simulink model "test_loopback_buf"  (Simulink 6.2)
settings: Solver=ode45  StartTime=0.0  StopTime=4000  RelTol=1e-3
undefined symbols (not defined in the file): Down, Up
libraries: xbsIndex_r3 x1383, xps_library x52, casper_library x37
(part 4 of 8)

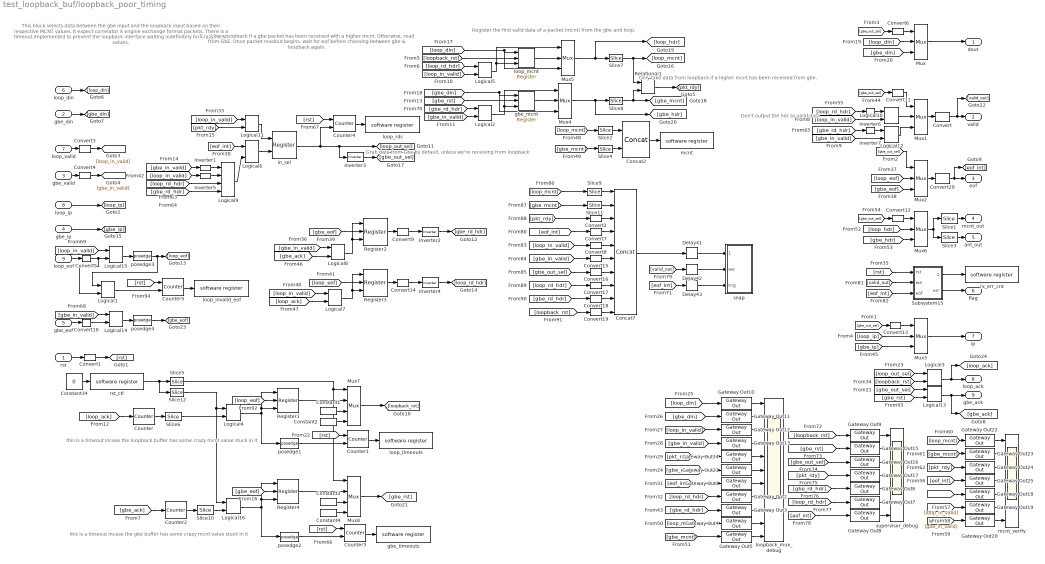
== system test_loopback_buf/loopback_poor_timing ==
  note: Read from loopback if a gbe packet
      | has been received with a higher mcnt.
      | Otherwise, read from GbE.
      | Once packet readout begins, wait for eof
      | before choosing between gbe & loopback again.
  note: Only take data from loopback
      | if a higher mcnt has been
      | received from gbe.
  note: This block selects data between the gbe input
      | and the loopback input based on their respective MCNT values.
      | It expect correlator X engine exchange format packets.
      |
      | There is a timeout implemented to prevent the loopback interface
      | waiting indefinitely for crazy MCNT values.
  note: Don't output the hdr
      | as valid data
  note: this is a timeout incase
      | the gbe buffer has
      | some crazy mcnt value stuck in it
  note: this is a timeout incase
      | the loopback buffer has
      | some crazy mcnt value stuck in it
  note: Grab data from
      | Gbe by default,
      | unless we're receiving
      | from loopback
  note: Register the first valid
      | data of a packet (mcnt)
      | from the gbe and loop.
  rst : Inport  Port=1  LatchInput=off
  gbe_din : Inport  Port=2  LatchInput=off
  gbe_valid : Inport  Port=3  LatchInput=off
  gbe_ip : Inport  Port=4  LatchInput=off
  gbe_eof : Inport  Port=5  LatchInput=off
  loop_din : Inport  Port=6  LatchInput=off
  loop_valid : Inport  Port=7  LatchInput=off
  loop_ip : Inport  Port=8  LatchInput=off
  loop_eof : Inport  Port=9  LatchInput=off
  Concat2 : xbsIndex_r3/Concat  num_inputs=2  explicit_period=off  period=1  dbl_ovrd=off
  Concat7 : xbsIndex_r3/Concat  num_inputs=10  explicit_period=off  period=1  dbl_ovrd=off
  Constant1 : xbsIndex_r3/Constant  const=0  equ=P=C  arith_type=Boolean  n_bits=1  bin_pt=0  opselect=C  inp2=PCIN>>17  opr=+  inp1=P  carry=CIN  iostate=0  explicit_period=on  period=1  dbl_ovrd=off
  Constant2 : xbsIndex_r3/Constant  const=1  equ=P=C  arith_type=Boolean  n_bits=1  bin_pt=0  opselect=C  inp2=PCIN>>17  opr=+  inp1=P  carry=CIN  iostate=0  explicit_period=on  period=1  dbl_ovrd=off
  Constant3 : xbsIndex_r3/Constant  const=0  equ=P=C  arith_type=Boolean  n_bits=1  bin_pt=0  opselect=C  inp2=PCIN>>17  opr=+  inp1=P  carry=CIN  iostate=0  explicit_period=on  period=1  dbl_ovrd=off
  Constant34 : Constant  Value=0
  Constant4 : xbsIndex_r3/Constant  const=1  equ=P=C  arith_type=Boolean  n_bits=1  bin_pt=0  opselect=C  inp2=PCIN>>17  opr=+  inp1=P  carry=CIN  iostate=0  explicit_period=on  period=1  dbl_ovrd=off
  Convert{,1,9,14,20} (5 alike) : xbsIndex_r3/Convert  arith_type=Boolean  n_bits=8  bin_pt=6  quantization=Truncate  overflow=Wrap  latency=0  explicit_period=off  period=1  dbl_ovrd=off  show_param=off  inserted_by_tool=off  pipeline=off
      settings: xl_area=[0, 0, 0, 0, 0, 0, 0]
  Convert{3..5,10} (4 alike) : xbsIndex_r3/Convert  arith_type=Boolean  n_bits=1  bin_pt=0  quantization=Truncate  overflow=Wrap  latency=0  explicit_period=on  period=1  dbl_ovrd=off  show_param=off  inserted_by_tool=off  pipeline=off
      settings: xl_area=[0, 0, 0, 0, 0, 0, 0]
  Convert{2,6..8,11..13,15..19} (12 alike) : xbsIndex_r3/Convert  arith_type=Unsigned  n_bits=1  bin_pt=0  quantization=Truncate  overflow=Wrap  latency=0  explicit_period=off  period=1  dbl_ovrd=off  show_param=off  inserted_by_tool=off  pipeline=off
      settings: xl_area=[0, 0, 0, 0, 0, 0, 0]
  Counter : xbsIndex_r3/Counter  cnt_type=Free Running  n_bits=timeout_bits+1  bin_pt=0  arith_type=Unsigned  start_count=0  cnt_to=Inf  cnt_by_val=1  operation=Up  explicit_period=off  period=1  load_pin=off  rst=on  en=off  dbl_ovrd=off  show_param=off  use_rpm=on  gen_core=off
      settings: xl_area=[0, 0, 0, 0, 0, 0, 0]
  Counter{1,3..5} (4 alike) : xbsIndex_r3/Counter  cnt_type=Free Running  n_bits=27  bin_pt=0  arith_type=Unsigned  start_count=0  cnt_to=Inf  cnt_by_val=1  operation=Up  explicit_period=off  period=1  load_pin=off  rst=on  en=on  dbl_ovrd=off  show_param=off  use_rpm=on  gen_core=off
      settings: xl_area=[0, 0, 0, 0, 0, 0, 0]
  Counter2 : xbsIndex_r3/Counter  cnt_type=Free Running  n_bits=timeout_bits+1  bin_pt=0  arith_type=Unsigned  start_count=0  cnt_to=Inf  cnt_by_val=1  operation=Up  explicit_period=off  period=1  load_pin=off  rst=on  en=off  dbl_ovrd=off  show_param=off  use_rpm=on  gen_core=off
      settings: xl_area=[0, 0, 0, 0, 0, 0, 0]
  Delay41 : xbsIndex_r3/Delay  latency=2  reg_retiming=on  explicit_period=on  period=1  en=off  accept_only_valid=off  init_zero=on  dbl_ovrd=off  show_param=off
      settings: xl_area=[0, 0, 0, 0, 0, 0, 0]
  Delay42 : xbsIndex_r3/Delay  latency=2  reg_retiming=on  explicit_period=on  period=1  en=off  accept_only_valid=off  init_zero=on  dbl_ovrd=off  show_param=off
      settings: xl_area=[0, 0, 0, 0, 0, 0, 0]
  Delay43 : xbsIndex_r3/Delay  latency=2  reg_retiming=on  explicit_period=on  period=1  en=off  accept_only_valid=off  init_zero=on  dbl_ovrd=off  show_param=off
      settings: xl_area=[0, 0, 0, 0, 0, 0, 0]
  Gateway Out{1..25} (25 alike) : xbsIndex_r3/Gateway Out  output_type=Double  nbits=8  bin_pt=6  arith_type=Boolean  quantization=Truncate  overflow=Wrap  hdl_port=on  timing_constraint=None  locs_specified=off  LOCs={}  needs_fixed_name=off  show_param=off
      settings: xl_area=[0, 0, 0, 0, 0, 0, 0]
  Inverter{1..7} (7 alike) : xbsIndex_r3/Inverter  latency=0  explicit_period=off  period=1  en=off  dbl_ovrd=off  show_param=off
      settings: xl_area=[0, 0, 0, 0, 0, 0, 0]
  Logical1 : xbsIndex_r3/Logical  logical_function=XOR  inputs=2  precision=Full  arith_type=Unsigned  n_bits=8  bin_pt=2  align_bp=on  latency=0  explicit_period=on  period=1  en=off  dbl_ovrd=off  show_param=off
      settings: xl_area=[0, 0, 0, 0, 0, 0, 0]
  Logical{7..8,10,14..15} (5 alike) : xbsIndex_r3/Logical  logical_function=AND  inputs=2  precision=Full  arith_type=Unsigned  n_bits=8  bin_pt=2  align_bp=on  latency=0  explicit_period=on  period=1  en=off  dbl_ovrd=off  show_param=off
      settings: xl_area=[0, 0, 0, 0, 0, 0, 0]
  Logical{2,5,11..12} (4 alike) : xbsIndex_r3/Logical  logical_function=AND  inputs=2  precision=Full  arith_type=Unsigned  n_bits=8  bin_pt=2  align_bp=on  latency=0  explicit_period=off  period=1  en=off  dbl_ovrd=off  show_param=off
      settings: xl_area=[0, 0, 0, 0, 0, 0, 0]
  Logical13 : xbsIndex_r3/Logical  logical_function=OR  inputs=2  precision=Full  arith_type=Unsigned  n_bits=8  bin_pt=2  align_bp=on  latency=0  explicit_period=off  period=1  en=off  dbl_ovrd=off  show_param=off
      settings: xl_area=[0, 0, 0, 0, 0, 0, 0]
  Logical16 : xbsIndex_r3/Logical  logical_function=OR  inputs=2  precision=Full  arith_type=Unsigned  n_bits=8  bin_pt=2  align_bp=on  latency=0  explicit_period=on  period=1  en=off  dbl_ovrd=off  show_param=off
      settings: xl_area=[0, 0, 0, 0, 0, 0, 0]
  Logical3 : xbsIndex_r3/Logical  logical_function=OR  inputs=2  precision=Full  arith_type=Unsigned  n_bits=8  bin_pt=2  align_bp=on  latency=0  explicit_period=off  period=1  en=off  dbl_ovrd=off  show_param=off
      settings: xl_area=[0, 0, 0, 0, 0, 0, 0]
  Logical4 : xbsIndex_r3/Logical  logical_function=OR  inputs=2  precision=Full  arith_type=Unsigned  n_bits=8  bin_pt=2  align_bp=on  latency=0  explicit_period=on  period=1  en=off  dbl_ovrd=off  show_param=off
      settings: xl_area=[0, 0, 0, 0, 0, 0, 0]
  Logical6 : xbsIndex_r3/Logical  logical_function=OR  inputs=2  precision=Full  arith_type=Unsigned  n_bits=8  bin_pt=2  align_bp=on  latency=0  explicit_period=off  period=1  en=off  dbl_ovrd=off  show_param=off
      settings: xl_area=[0, 0, 0, 0, 0, 0, 0]
  Logical9 : xbsIndex_r3/Logical  logical_function=AND  inputs=4  precision=Full  arith_type=Unsigned  n_bits=8  bin_pt=2  align_bp=on  latency=0  explicit_period=on  period=1  en=off  dbl_ovrd=off  show_param=off
      settings: xl_area=[0, 0, 0, 0, 0, 0, 0]
  Mux{,1,3..6} (6 alike) : xbsIndex_r3/Mux  inputs=2  precision=Full  arith_type="Signed  (2's comp)"  n_bits=8  bin_pt=2  quantization=Truncate  overflow=Wrap  latency=0  explicit_period=off  period=1  en=off  dbl_ovrd=off  show_param=off  mux_type=off  use_rpm=off  gen_core=off
      settings: xl_area=[0, 0, 0, 0, 0, 0, 0]
  Mux2 : xbsIndex_r3/Mux  inputs=2  precision=Full  arith_type="Signed  (2's comp)"  n_bits=8  bin_pt=2  quantization=Truncate  overflow=Wrap  latency=0  explicit_period=on  period=1  en=off  dbl_ovrd=off  show_param=off  mux_type=off  use_rpm=off  gen_core=off
      settings: xl_area=[0, 0, 0, 0, 0, 0, 0]
  Mux7 : xbsIndex_r3/Mux  inputs=3  precision=Full  arith_type="Signed  (2's comp)"  n_bits=8  bin_pt=2  quantization=Truncate  overflow=Wrap  latency=0  explicit_period=off  period=1  en=off  dbl_ovrd=off  show_param=off  mux_type=off  use_rpm=off  gen_core=off
      settings: xl_area=[0, 0, 0, 0, 0, 0, 0]
  Mux8 : xbsIndex_r3/Mux  inputs=3  precision=Full  arith_type="Signed  (2's comp)"  n_bits=8  bin_pt=2  quantization=Truncate  overflow=Wrap  latency=0  explicit_period=off  period=1  en=off  dbl_ovrd=off  show_param=off  mux_type=off  use_rpm=off  gen_core=off
      settings: xl_area=[0, 0, 0, 0, 0, 0, 0]
  Register{1..4} (4 alike) : xbsIndex_r3/Register  init=0  reg_only_valid=off  explicit_period=on  period=1  rst=on  en=on  out_en=off  dbl_ovrd=off  show_param=off
      settings: xl_area=[0, 0, 0, 0, 0, 0, 0]
  Relational1 : xbsIndex_r3/Relational  mode=a<b  latency=0  explicit_period=off  period=1  en=off  dbl_ovrd=off  show_param=off
      settings: xl_area=[0, 0, 0, 0, 0, 0, 0]
  Slice1 : xbsIndex_r3/Slice  mode=Lower Bit Location + Width  nbits=48  bit1=0  base1=MSB of Input  bit0=16  base0=LSB of Input  boolean_output=off  explicit_period=off  period=1  dbl_ovrd=off
  Slice10 : xbsIndex_r3/Slice  mode=Upper Bit Location + Width  nbits=1  bit1=0  base1=MSB of Input  bit0=1  base0=LSB of Input  boolean_output=on  explicit_period=off  period=1  dbl_ovrd=off
  Slice11 : xbsIndex_r3/Slice  mode=Lower Bit Location + Width  nbits=12  bit1=0  base1=MSB of Input  bit0=0  base0=LSB of Input  boolean_output=off  explicit_period=off  period=1  dbl_ovrd=off
  Slice12 : xbsIndex_r3/Slice  mode=Lower Bit Location + Width  nbits=1  bit1=0  base1=MSB of Input  bit0=0  base0=LSB of Input  boolean_output=on  explicit_period=off  period=1  dbl_ovrd=off
  Slice2 : xbsIndex_r3/Slice  mode=Lower Bit Location + Width  nbits=16  bit1=0  base1=MSB of Input  bit0=0  base0=LSB of Input  boolean_output=off  explicit_period=off  period=1  dbl_ovrd=off
  Slice3 : xbsIndex_r3/Slice  mode=Lower Bit Location + Width  nbits=16  bit1=0  base1=MSB of Input  bit0=0  base0=LSB of Input  boolean_output=off  explicit_period=off  period=1  dbl_ovrd=off
  Slice4 : xbsIndex_r3/Slice  mode=Lower Bit Location + Width  nbits=16  bit1=0  base1=MSB of Input  bit0=0  base0=LSB of Input  boolean_output=off  explicit_period=off  period=1  dbl_ovrd=off
  Slice5 : xbsIndex_r3/Slice  mode=Lower Bit Location + Width  nbits=2  bit1=0  base1=MSB of Input  bit0=1  base0=LSB of Input  boolean_output=off  explicit_period=off  period=1  dbl_ovrd=off
  Slice6 : xbsIndex_r3/Slice  mode=Upper Bit Location + Width  nbits=1  bit1=0  base1=MSB of Input  bit0=1  base0=LSB of Input  boolean_output=on  explicit_period=off  period=1  dbl_ovrd=off
  Slice7 : xbsIndex_r3/Slice  mode=Upper Bit Location + Width  nbits=48  bit1=0  base1=MSB of Input  bit0=0  base0=LSB of Input  boolean_output=off  explicit_period=off  period=1  dbl_ovrd=off
  Slice8 : xbsIndex_r3/Slice  mode=Upper Bit Location + Width  nbits=48  bit1=0  base1=MSB of Input  bit0=0  base0=LSB of Input  boolean_output=off  explicit_period=off  period=1  dbl_ovrd=off
  Slice9 : xbsIndex_r3/Slice  mode=Lower Bit Location + Width  nbits=12  bit1=0  base1=MSB of Input  bit0=0  base0=LSB of Input  boolean_output=off  explicit_period=off  period=1  dbl_ovrd=off
  Subsystem15 : Subsystem  mask{payload_len=payload_len}
      mask init:
      | fmtstr = sprintf('Payload Length: %d', payload_len);
      | set_param(gcb, 'AttributesFormatString', fmtstr);
      settings: AttributesFormatString=Payload Length: 50
  gbe_mcnt : xbsIndex_r3/Register  init=0  reg_only_valid=off  explicit_period=on  period=1  rst=on  en=on  out_en=off  dbl_ovrd=off  show_param=off
      settings: xl_area=[0, 0, 0, 0, 0, 0, 0]
  gbe_timeouts : xps_library/software register  Tag=xps:sw_reg  io_dir=To Processor  arith_type=Unsigned  bitwidth=32  bin_pt=0  sample_period=1  gw_name=test_loopback_buf_loopback_poor_timing_gbe_timeouts_user_data_in
  in_sel : xbsIndex_r3/Register  init=0  reg_only_valid=off  explicit_period=on  period=1  rst=off  en=on  out_en=off  dbl_ovrd=off  show_param=off
      settings: xl_area=[0, 0, 0, 0, 0, 0, 0]
  loop_invalid_eof : xps_library/software register  Tag=xps:sw_reg  io_dir=To Processor  arith_type=Unsigned  bitwidth=32  bin_pt=0  sample_period=1  gw_name=test_loopback_buf_loopback_poor_timing_loop_invalid_eof_user_data_in
  loop_mcnt : xbsIndex_r3/Register  init=0  reg_only_valid=off  explicit_period=on  period=1  rst=on  en=on  out_en=off  dbl_ovrd=off  show_param=off
      settings: xl_area=[0, 0, 0, 0, 0, 0, 0]
  loop_rds : xps_library/software register  Tag=xps:sw_reg  io_dir=To Processor  arith_type=Unsigned  bitwidth=32  bin_pt=0  sample_period=1  gw_name=test_loopback_buf_loopback_poor_timing_loop_rds_user_data_in
  loop_timeouts : xps_library/software register  Tag=xps:sw_reg  io_dir=To Processor  arith_type=Unsigned  bitwidth=32  bin_pt=0  sample_period=1  gw_name=test_loopback_buf_loopback_poor_timing_loop_timeouts_user_data_in
  loopback_mux_debug : Scope  NumInputPorts=11
      settings: YMin=300~190.95~0~0.95~0.95~-1~-1~-1~-5~-5~-5  YMax=525~211.05~1~1.05~1.05~1~1~1~5~5~5  SaveName=ScopeData7
  mcnt : xps_library/software register  Tag=xps:sw_reg  io_dir=To Processor  arith_type=Unsigned  bitwidth=32  bin_pt=0  sample_period=1  gw_name=test_loopback_buf_loopback_poor_timing_mcnt_user_data_in
  mcnt_verify : Scope  NumInputPorts=7
      settings: YMin=300~190.95~0~-5~-5~-5~-5  YMax=525~211.05~1~5~5~5~5  SaveName=ScopeData2
  posedge{1..4} (4 alike) : casper_library/Misc/posedge  Tag=Rising Edge Detector
  rst_ctl : xps_library/software register  Tag=xps:sw_reg  io_dir=From Processor  arith_type=Unsigned  bitwidth=32  bin_pt=0  sample_period=1  gw_name=test_loopback_buf_loopback_poor_timing_rst_ctl_user_data_out
  rx_err_cnt : xps_library/software register  Tag=xps:sw_reg  io_dir=To Processor  arith_type=Unsigned  bitwidth=32  bin_pt=0  sample_period=1  gw_name=test_loopback_buf_loopback_poor_timing_rx_err_cnt_user_data_in
  snap : Subsystem  mask{nsamples=12}
      mask prompts: nsamples "Number of Samples (2^?)"
  supervisor_debug : Scope  NumInputPorts=7
      settings: YMin=300~190.95~0~-5~-5~-5~-5  YMax=525~211.05~1~5~5~5~5  SaveName=ScopeData18
  dout : Outport
  valid : Outport  Port=2
  eof : Outport  Port=3
  mcnt_out : Outport  Port=4
  ant_out : Outport  Port=5
  flag : Outport  Port=6
  ip : Outport  Port=7
  loop_ack : Outport  Port=8
  gbe_ack : Outport  Port=9
  wires:
  Mux/1 -> dout/1
  Mux1/1 -> Convert/1
  Mux2/1 -> Convert20/1
  gbe_valid/1 -> Convert4/1
  loop_valid/1 -> Convert3/1
  Convert/1 -> valid/1, [valid_out]
  Slice2/1 -> Concat2/1
  Slice4/1 -> Concat2/2
  Concat2/1 -> mcnt/1
  Convert6/1 -> Mux/1
  [gbe_out_sel] -> Convert6/1
  [gbe_out_sel] -> Mux2/1
  Gateway Out12/1 -> loopback_mux_debug/3
  Gateway Out13/1 -> loopback_mux_debug/4
  Gateway Out14/1 -> loopback_mux_debug/5
  Gateway Out21/1 -> loopback_mux_debug/6
  Convert3/1 -> [loop_in_valid]
  Convert4/1 -> [gbe_in_valid]
  Relational1/1 -> [pkt_rdy]
  loop_din/1 -> [loop_din]
  gbe_din/1 -> [gbe_din]
  [loop_din] -> Mux/2
  [gbe_din] -> Mux/3
  [gbe_din] -> Gateway Out11/1
  [loop_din] -> Gateway Out10/1
  [loop_in_valid] -> Gateway Out12/1
  [gbe_in_valid] -> Gateway Out13/1
  [gbe_out_sel] -> Gateway Out21/1
  [pkt_rdy] -> Gateway Out14/1
  Gateway Out1/1 -> loopback_mux_debug/7
  [eof_int] -> Gateway Out1/1
  [loop_rd_hdr] -> Gateway Out2/1
  Gateway Out2/1 -> loopback_mux_debug/8
  [loop_eof] -> Mux2/2
  loop_eof/1 -> Convert5/1
  gbe_eof/1 -> Convert10/1
  [gbe_eof] -> Mux2/3
  Gateway Out3/1 -> loopback_mux_debug/9
  [gbe_rd_hdr] -> Gateway Out3/1
  [gbe_out_sel] -> Convert11/1
  Convert11/1 -> Mux1/1
  loop_ip/1 -> [loop_ip]
  gbe_ip/1 -> [gbe_ip]
  Mux3/1 -> ip/1
  [loop_ip] -> Mux3/2
  [gbe_ip] -> Mux3/3
  [gbe_out_sel] -> Convert13/1
  Convert13/1 -> Mux3/1
  [loop_mcnt] -> Slice2/1
  [gbe_mcnt] -> Slice4/1
  Gateway Out10/1 -> loopback_mux_debug/1
  Gateway Out11/1 -> loopback_mux_debug/2
  Gateway Out4/1 -> loopback_mux_debug/10
  Gateway Out5/1 -> loopback_mux_debug/11
  [loop_mcnt] -> Gateway Out4/1
  [gbe_mcnt] -> Gateway Out5/1
  Gateway Out24/1 -> mcnt_verify/3
  Gateway Out22/1 -> mcnt_verify/1
  Gateway Out23/1 -> mcnt_verify/2
  Gateway Out25/1 -> mcnt_verify/4
  Gateway Out18/1 -> mcnt_verify/5
  Gateway Out19/1 -> mcnt_verify/6
  Gateway Out20/1 -> mcnt_verify/7
  [gbe_out_sel] -> Gateway Out20/1
  [gbe_in_valid] -> Gateway Out19/1
  [loop_in_valid] -> Gateway Out18/1
  [eof_int] -> Gateway Out25/1
  [loop_mcnt] -> Gateway Out22/1
  [gbe_mcnt] -> Gateway Out23/1
  [pkt_rdy] -> Gateway Out24/1
  Mux4/1 -> Slice8/1, [gbe_hdr]
  Mux5/1 -> Slice7/1, [loop_hdr]
  Slice7/1 -> Relational1/1, [loop_mcnt]
  Slice8/1 -> Relational1/2, [gbe_mcnt]
  Slice1/1 -> mcnt_out/1
  Slice3/1 -> ant_out/1
  Convert12/1 -> Mux6/1
  [gbe_out_sel] -> Convert12/1
  [loop_hdr] -> Mux6/2
  [gbe_hdr] -> Mux6/3
  Mux6/1 -> Slice1/1, Slice3/1
  Inverter6/1 -> Logical10/1
  Logical10/1 -> Mux1/2
  [loop_in_valid] -> Logical10/2
  [loop_rd_hdr] -> Inverter6/1
  [gbe_rd_hdr] -> Inverter7/1
  [gbe_in_valid] -> Logical12/2
  Logical12/1 -> Mux1/3
  Inverter7/1 -> Logical12/1
  Counter2/1 -> Slice10/1
  [gbe_ack] -> Counter2/1
  [rst] -> Counter3/1
  Counter3/1 -> gbe_timeouts/1
  Logical16/1 -> Register4/1, Register4/3, posedge2/1
  Logical14/1 -> posedge4/1
  Logical15/1 -> posedge3/1
  Convert5/1 -> Logical15/2, Logical1/2
  Convert10/1 -> Logical14/2
  [gbe_in_valid] -> Logical14/1
  [loop_in_valid] -> Logical15/1
  Slice10/1 -> Logical16/2
  Gateway Out16/1 -> supervisor_debug/3
  Gateway Out9/1 -> supervisor_debug/1
  Gateway Out15/1 -> supervisor_debug/2
  Gateway Out17/1 -> supervisor_debug/4
  Gateway Out6/1 -> supervisor_debug/5
  Gateway Out7/1 -> supervisor_debug/6
  Gateway Out8/1 -> supervisor_debug/7
  [loopback_rst] -> Gateway Out9/1
  [gbe_rst] -> Gateway Out15/1
  [gbe_out_sel] -> Gateway Out16/1
  [pkt_rdy] -> Gateway Out17/1
  [gbe_rd_hdr] -> Gateway Out6/1
  [loop_rd_hdr] -> Gateway Out7/1
  [eof_int] -> Gateway Out8/1
  Logical3/1 -> loop_ack/1, [loop_ack]
  Logical13/1 -> gbe_ack/1, [gbe_ack]
  rst/1 -> Convert1/1
  Subsystem15/1(err_cnt) -> rx_err_cnt/1
  Subsystem15/2(err) -> flag/1
  [rst] -> Subsystem15/1(rst)
  [valid_out] -> Subsystem15/2(we)
  [eof_int] -> Subsystem15/3(eof)
  Counter/1 -> Slice6/1
  Slice6/1 -> Logical4/2
  [loop_ack] -> Counter/1
  [rst] -> Counter1/1
  Counter1/1 -> loop_timeouts/1
  Logical4/1 -> Register1/1, Register1/3, posedge1/1
  [pkt_rdy] -> Logical11/2
  [eof_int] -> Logical6/1
  Inverter3/1 -> [gbe_out_sel]
  in_sel/1 -> Inverter3/1, [loop_out_sel], Counter4/2
  Logical6/1 -> in_sel/2
  [loop_in_valid] -> Logical11/1
  Register2/1 -> Convert9/1
  Convert9/1 -> Inverter2/1
  Inverter2/1 -> [gbe_rd_hdr]
  [gbe_eof] -> Register2/2
  Register3/1 -> Convert14/1
  Convert14/1 -> Inverter4/1
  Inverter4/1 -> [loop_rd_hdr]
  [loop_eof] -> Register3/2
  Logical11/1 -> in_sel/1
  Logical8/1 -> Register2/1, Register2/3
  [gbe_in_valid] -> Logical8/1
  [gbe_ack] -> Logical8/2
  Logical7/1 -> Register3/1, Register3/3
  [loop_in_valid] -> Logical7/1
  [loop_ack] -> Logical7/2
  [gbe_in_valid] -> Inverter1/1
  [loop_in_valid] -> Inverter5/1
  Logical9/1 -> Logical6/2
  Inverter1/1 -> Logical9/1
  Inverter5/1 -> Logical9/2
  [loop_rd_hdr] -> Logical9/3
  [gbe_rd_hdr] -> Logical9/4
  gbe_mcnt/1 -> Mux4/2
  loop_mcnt/1 -> Mux5/2
  Logical2/1 -> gbe_mcnt/3, Mux4/1
  Logical5/1 -> Mux5/1, loop_mcnt/3
  [loop_rd_hdr] -> Logical5/1
  [gbe_rd_hdr] -> Logical2/1
  [loop_in_valid] -> Logical5/2
  [gbe_in_valid] -> Logical2/2
  [loop_din] -> loop_mcnt/1, Mux5/3
  [gbe_din] -> gbe_mcnt/1, Mux4/3
  Concat7/1 -> Delay41/1
  Delay42/1 -> snap/2(we)
  Delay43/1 -> snap/3(trig)
  Delay41/1 -> snap/1(data_in)
  [valid_out] -> Delay42/1
  [eof_int] -> Delay43/1
  [loop_mcnt] -> Slice9/1
  [gbe_mcnt] -> Slice11/1
  Slice9/1 -> Concat7/1
  Slice11/1 -> Concat7/2
  [pkt_rdy] -> Convert2/1
  [eof_int] -> Convert7/1
  [loop_in_valid] -> Convert8/1
  [gbe_in_valid] -> Convert15/1
  [gbe_out_sel] -> Convert16/1
  [loop_rd_hdr] -> Convert17/1
  [gbe_rd_hdr] -> Convert18/1
  [loopback_rst] -> Convert19/1
  [loop_eof] -> Register1/2
  [gbe_eof] -> Register4/2
  [loop_out_sel] -> Logical3/1
  [gbe_out_sel] -> Logical13/1
  [loopback_rst] -> Logical3/2
  [gbe_rst] -> Logical13/2
  Mux7/1 -> [loopback_rst]
  Register1/1 -> Mux7/2
  Mux8/1 -> [gbe_rst]
  Register4/1 -> Mux8/2
  Constant1/1 -> Mux7/3
  Constant34/1 -> rst_ctl/1
  rst_ctl/1 -> Slice5/1, Slice12/1
  Slice5/1 -> Mux7/1, Mux8/1
  Convert1/1 -> [rst]
  Slice12/1 -> Logical4/1, Logical16/1
  [loopback_rst] -> loop_mcnt/2
  [gbe_rst] -> gbe_mcnt/2
  Convert2/1 -> Concat7/3
  Convert7/1 -> Concat7/4
  Convert8/1 -> Concat7/5
  Convert15/1 -> Concat7/6
  Convert16/1 -> Concat7/7
  Convert17/1 -> Concat7/8
  Convert18/1 -> Concat7/9
  Convert19/1 -> Concat7/10
  Counter4/1 -> loop_rds/1
  [rst] -> Counter4/1
  Convert20/1 -> [eof_int], eof/1
  posedge1/1 -> Counter1/2
  posedge2/1 -> Counter3/2
  posedge3/1 -> [loop_eof], Logical1/1
  posedge4/1 -> [gbe_eof]
  [rst] -> Counter5/1
  Counter5/1 -> loop_invalid_eof/1
  Logical1/1 -> Counter5/2
  Constant2/1 -> Mux7/4
  Constant3/1 -> Mux8/3
  Constant4/1 -> Mux8/4

== system test_loopback_buf/mux_pkts_orig ==
  note: Read from loopback if a gbe packet
      | has been received with a higher mcnt.
      | Otherwise, wait until gbe has one ready.
      | Once packet readout begins, wait for eof
      | before choosing between gbe & loopback again.
  note: Register the first valid
      | data of a packet (mcnt)
      | from the gbe.
  note: Only take data from loopback
      | if a higher mcnt has been
      | received from gbe.
  gbe_din : Inport  Port=1  LatchInput=off
  gbe_valid : Inport  Port=2  LatchInput=off
  gbe_eof : Inport  Port=3  LatchInput=off
  loop_din : Inport  Port=4  LatchInput=off
  loop_valid : Inport  Port=5  LatchInput=off
  loop_eof : Inport  Port=6  LatchInput=off
  Concat2 : xbsIndex_r3/Concat  num_inputs=2  explicit_period=off  period=1  dbl_ovrd=off
  Constant1 : Constant  Value=0
  Convert : xbsIndex_r3/Convert  arith_type=Boolean  n_bits=8  bin_pt=6  quantization=Truncate  overflow=Wrap  latency=0  explicit_period=off  period=1  dbl_ovrd=off  show_param=off  inserted_by_tool=off  pipeline=off
      settings: xl_area=[0, 0, 0, 0, 0, 0, 0]
  Convert1 : xbsIndex_r3/Convert  arith_type=Boolean  n_bits=8  bin_pt=6  quantization=Truncate  overflow=Wrap  latency=0  explicit_period=off  period=1  dbl_ovrd=off  show_param=off  inserted_by_tool=off  pipeline=off
      settings: xl_area=[0, 0, 0, 0, 0, 0, 0]
  Convert2 : xbsIndex_r3/Convert  arith_type=Boolean  n_bits=8  bin_pt=6  quantization=Truncate  overflow=Wrap  latency=0  explicit_period=off  period=1  dbl_ovrd=off  show_param=off  inserted_by_tool=off  pipeline=off
      settings: xl_area=[0, 0, 0, 0, 0, 0, 0]
  Convert{4..5,7..8} (4 alike) : xbsIndex_r3/Convert  arith_type=Boolean  n_bits=1  bin_pt=0  quantization=Truncate  overflow=Wrap  latency=0  explicit_period=on  period=1  dbl_ovrd=off  show_param=off  inserted_by_tool=off  pipeline=off
      settings: xl_area=[0, 0, 0, 0, 0, 0, 0]
  Convert6 : xbsIndex_r3/Convert  arith_type=Unsigned  n_bits=1  bin_pt=0  quantization=Truncate  overflow=Wrap  latency=0  explicit_period=off  period=1  dbl_ovrd=off  show_param=off  inserted_by_tool=off  pipeline=off
      settings: xl_area=[0, 0, 0, 0, 0, 0, 0]
  Delay1 : xbsIndex_r3/Delay  latency=1  reg_retiming=off  explicit_period=off  period=1  en=off  accept_only_valid=off  init_zero=on  dbl_ovrd=off  show_param=off
      settings: xl_area=[0, 0, 0, 0, 0, 0, 0]
  Inverter2 : xbsIndex_r3/Inverter  Orientation=left  latency=0  explicit_period=off  period=1  en=off  dbl_ovrd=off  show_param=off
      settings: xl_area=[0, 0, 0, 0, 0, 0, 0]
  Logical : xbsIndex_r3/Logical  logical_function=OR  inputs=2  precision=Full  arith_type=Unsigned  n_bits=8  bin_pt=2  align_bp=on  latency=0  explicit_period=off  period=1  en=off  dbl_ovrd=off  show_param=off
      settings: xl_area=[0, 0, 0, 0, 0, 0, 0]
  Logical{1..5,7..8} (7 alike) : xbsIndex_r3/Logical  logical_function=AND  inputs=2  precision=Full  arith_type=Unsigned  n_bits=8  bin_pt=2  align_bp=on  latency=0  explicit_period=off  period=1  en=off  dbl_ovrd=off  show_param=off
      settings: xl_area=[0, 0, 0, 0, 0, 0, 0]
  Logical9 : xbsIndex_r3/Logical  logical_function=OR  inputs=2  precision=Full  arith_type=Unsigned  n_bits=8  bin_pt=2  align_bp=on  latency=1  explicit_period=off  period=1  en=off  dbl_ovrd=off  show_param=off
      settings: xl_area=[0, 0, 0, 0, 0, 0, 0]
  Mux : xbsIndex_r3/Mux  inputs=2  precision=Full  arith_type="Signed  (2's comp)"  n_bits=8  bin_pt=2  quantization=Truncate  overflow=Wrap  latency=1  explicit_period=off  period=1  en=off  dbl_ovrd=off  show_param=off  mux_type=off  use_rpm=off  gen_core=off
      settings: xl_area=[0, 0, 0, 0, 0, 0, 0]
  Mux2 : xbsIndex_r3/Mux  inputs=2  precision=Full  arith_type="Signed  (2's comp)"  n_bits=8  bin_pt=2  quantization=Truncate  overflow=Wrap  latency=0  explicit_period=off  period=1  en=off  dbl_ovrd=off  show_param=off  mux_type=off  use_rpm=off  gen_core=off
      settings: xl_area=[0, 0, 0, 0, 0, 0, 0]
  Relational1 : xbsIndex_r3/Relational  mode=a<=b  latency=1  explicit_period=off  period=1  en=off  dbl_ovrd=off  show_param=off
      settings: xl_area=[0, 0, 0, 0, 0, 0, 0]
  Slice : xbsIndex_r3/Slice  mode=Lower Bit Location + Width  nbits=1  bit1=0  base1=MSB of Input  bit0=1  base0=LSB of Input  boolean_output=off  explicit_period=off  period=1  dbl_ovrd=off
  Slice1 : xbsIndex_r3/Slice  mode=Upper Bit Location + Width  nbits=48  bit1=0  base1=MSB of Input  bit0=0  base0=LSB of Input  boolean_output=off  explicit_period=off  period=1  dbl_ovrd=off
  Slice2 : xbsIndex_r3/Slice  mode=Lower Bit Location + Width  nbits=16  bit1=0  base1=MSB of Input  bit0=0  base0=LSB of Input  boolean_output=off  explicit_period=off  period=1  dbl_ovrd=off
  Slice3 : xbsIndex_r3/Slice  mode=Upper Bit Location + Width  nbits=48  bit1=0  base1=MSB of Input  bit0=0  base0=LSB of Input  boolean_output=off  explicit_period=off  period=1  dbl_ovrd=off
  Slice4 : xbsIndex_r3/Slice  mode=Lower Bit Location + Width  nbits=16  bit1=0  base1=MSB of Input  bit0=0  base0=LSB of Input  boolean_output=off  explicit_period=off  period=1  dbl_ovrd=off
  Slice5 : xbsIndex_r3/Slice  mode=Lower Bit Location + Width  nbits=1  bit1=0  base1=MSB of Input  bit0=0  base0=LSB of Input  boolean_output=off  explicit_period=off  period=1  dbl_ovrd=off
  gbe_mcnt : xbsIndex_r3/Register  init=0  reg_only_valid=off  explicit_period=on  period=1  rst=on  en=on  out_en=off  dbl_ovrd=off  show_param=off
      settings: xl_area=[0, 0, 0, 0, 0, 0, 0]
  loop_mcnt : xbsIndex_r3/Register  init=0  reg_only_valid=off  explicit_period=on  period=1  rst=on  en=on  out_en=off  dbl_ovrd=off  show_param=off
      settings: xl_area=[0, 0, 0, 0, 0, 0, 0]
  mcnt : xps_library/software register  Tag=xps:sw_reg  io_dir=To Processor  arith_type=Unsigned  bitwidth=32  bin_pt=0  sample_period=1  gw_name=test_loopback_buf_mux_pkts_orig_mcnt_user_data_in
  posedge : casper_library/Misc/posedge  Tag=Rising Edge Detector
  rst_mcnt_regs : xps_library/software register  Tag=xps:sw_reg  io_dir=From Processor  arith_type=Unsigned  bitwidth=32  bin_pt=0  sample_period=1  gw_name=test_loopback_buf_mux_pkts_orig_rst_mcnt_regs_user_data_out
  state_mach : Subsystem
  dout : Outport
  valid : Outport  Port=2
  eof : Outport  Port=3
  loop_ack : Outport  Port=4
  gbe_ack : Outport  Port=5
  wires:
  Mux/1 -> dout/1
  Logical9/1 -> Convert/1
  Mux2/1 -> Delay1/1, state_mach/3(eof)
  Delay1/1 -> eof/1
  gbe_din/1 -> Mux/3, Slice1/1
  loop_din/1 -> Mux/2, Slice3/1
  gbe_valid/1 -> Convert8/1
  loop_valid/1 -> Convert4/1
  state_mach/1(gbe_ack) -> Mux2/1, Convert6/1, Logical8/1, Convert5/1
  gbe_eof/1 -> Logical1/2
  loop_eof/1 -> Logical4/2
  Logical4/1 -> Mux2/2
  Logical1/1 -> Mux2/3
  state_mach/2(loop_ack) -> Logical7/1, Convert7/1
  Convert/1 -> valid/1
  Slice1/1 -> gbe_mcnt/1
  state_mach/3(state) -> Inverter2/1
  Inverter2/1 -> Logical2/1, Logical5/1
  gbe_mcnt/1 -> Relational1/2, Slice4/1
  Relational1/1 -> Logical3/1
  loop_mcnt/1 -> Relational1/1, Slice2/1
  Slice3/1 -> loop_mcnt/1
  Slice2/1 -> Concat2/1
  Slice4/1 -> Concat2/2
  Concat2/1 -> mcnt/1
  Convert6/1 -> Mux/1
  Convert5/1 -> gbe_ack/1
  Convert7/1 -> loop_ack/1
  Convert4/1 -> Logical4/1, Logical3/2, Logical7/2, Logical5/2
  Convert8/1 -> Logical2/2, Logical1/1, state_mach/1(gbe_valid), Logical8/2
  Logical7/1 -> Logical9/1
  Logical8/1 -> Logical9/2
  Logical/1 -> state_mach/2(pkt_rdy)
  Logical3/1 -> Logical/1
  Logical2/1 -> gbe_mcnt/3
  Logical5/1 -> loop_mcnt/3
  Slice/1 -> Convert1/1
  Constant1/1 -> rst_mcnt_regs/1
  rst_mcnt_regs/1 -> Slice5/1, Slice/1
  Slice5/1 -> posedge/1
  posedge/1 -> Convert2/1
  Convert1/1 -> Logical/2
  Convert2/1 -> loop_mcnt/2, gbe_mcnt/2

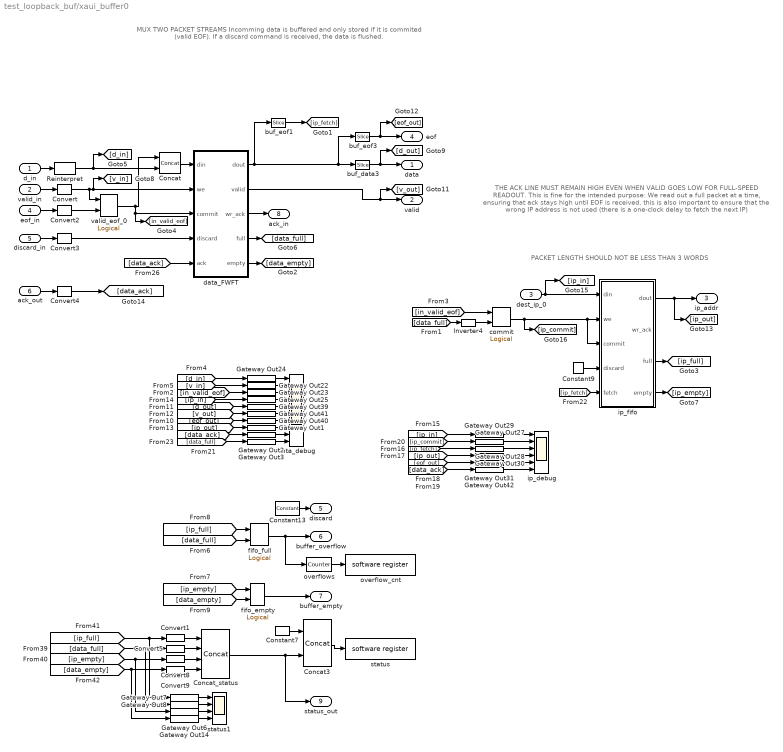
== system test_loopback_buf/xaui_buffer0 ==
  note: MUX TWO PACKET STREAMS
      | Incomming data is buffered and only stored if it is commited (valid EOF).
      | If a discard command is received, the data is flushed.
  note: THE ACK LINE MUST REMAIN HIGH EVEN WHEN VALID GOES LOW FOR FULL-SPEED READOUT.
      |
      | This is fine for the intended purpose:
      | We read out a full packet at a time, ensuring that ack stays high until EOF is received.
      |
      | this is also important to ensure that the wrong IP address is not used
      | (there is a one-clock delay to fetch the next IP)
  note: PACKET LENGTH SHOULD NOT BE LESS THAN 3 WORDS
  d_in : Inport  Port=1  LatchInput=off
  valid_in : Inport  Port=2  LatchInput=off
  dest_ip_0 : Inport  Port=3  LatchInput=off
  eof_in : Inport  Port=4  LatchInput=off
  discard_in : Inport  Port=5  LatchInput=off
  ack_out : Inport  Port=6  LatchInput=off
  Concat : xbsIndex_r3/Concat  num_inputs=2  explicit_period=off  period=1  dbl_ovrd=off
  Concat3 : xbsIndex_r3/Concat  num_inputs=2  explicit_period=off  period=1  dbl_ovrd=off
  Concat_status : xbsIndex_r3/Concat  num_inputs=4  explicit_period=on  period=1  dbl_ovrd=off
  Constant13 : xbsIndex_r3/Constant  const=0  equ=P=C  arith_type=Boolean  n_bits=1  bin_pt=0  opselect=C  inp2=PCIN>>17  opr=+  inp1=P  carry=CIN  iostate=0  explicit_period=on  period=1  dbl_ovrd=off
  Constant7 : xbsIndex_r3/Constant  const=0  equ=P=C  arith_type=Unsigned  n_bits=32-9  bin_pt=0  opselect=C  inp2=PCIN>>17  opr=+  inp1=P  carry=CIN  iostate=0  explicit_period=on  period=1  dbl_ovrd=off
  Constant9 : xbsIndex_r3/Constant  const=0  equ=P=C  arith_type=Boolean  n_bits=1  bin_pt=0  opselect=C  inp2=PCIN>>17  opr=+  inp1=P  carry=CIN  iostate=0  explicit_period=on  period=1  dbl_ovrd=off
  Convert{,2..4} (4 alike) : xbsIndex_r3/Convert  arith_type=Boolean  n_bits=8  bin_pt=6  quantization=Truncate  overflow=Wrap  latency=0  explicit_period=on  period=1  dbl_ovrd=off  show_param=off  inserted_by_tool=off  pipeline=off
      settings: xl_area=[0, 0, 0, 0, 0, 0, 0]
  Convert{1,5,8..9} (4 alike) : xbsIndex_r3/Convert  arith_type=Unsigned  n_bits=1  bin_pt=0  quantization=Truncate  overflow=Wrap  latency=0  explicit_period=off  period=1  dbl_ovrd=off  show_param=off  inserted_by_tool=off  pipeline=off
      settings: xl_area=[0, 0, 0, 0, 0, 0, 0]
  Gateway Out{1..3,6..8,14,22..25,27..31,39..42} (20 alike) : xbsIndex_r3/Gateway Out  output_type=Double  nbits=8  bin_pt=6  arith_type=Boolean  quantization=Truncate  overflow=Wrap  hdl_port=on  timing_constraint=None  locs_specified=off  LOCs={}  needs_fixed_name=off  show_param=off
      settings: xl_area=[0, 0, 0, 0, 0, 0, 0]
  Inverter4 : xbsIndex_r3/Inverter  latency=0  explicit_period=off  period=1  en=off  dbl_ovrd=off  show_param=off
      settings: xl_area=[0, 0, 0, 0, 0, 0, 0]
  Reinterpret : xbsIndex_r3/Reinterpret  force_arith_type=on  arith_type=Unsigned  force_bin_pt=on  bin_pt=0  force_valid=on
  buf_data3 : xbsIndex_r3/Slice  mode=Lower Bit Location + Width  nbits=64  bit1=33  base1=LSB of Input  bit0=0  base0=LSB of Input  boolean_output=off  explicit_period=off  period=1  dbl_ovrd=off
  buf_eof1 : xbsIndex_r3/Slice  mode=Upper Bit Location + Width  nbits=1  bit1=64  base1=LSB of Input  bit0=0  base0=LSB of Input  boolean_output=on  explicit_period=off  period=1  dbl_ovrd=off
  buf_eof3 : xbsIndex_r3/Slice  mode=Upper Bit Location + Width  nbits=1  bit1=64  base1=LSB of Input  bit0=0  base0=LSB of Input  boolean_output=on  explicit_period=off  period=1  dbl_ovrd=off
  commit : xbsIndex_r3/Logical  logical_function=AND  inputs=2  precision=Full  arith_type=Unsigned  n_bits=8  bin_pt=2  align_bp=on  latency=0  explicit_period=off  period=1  en=off  dbl_ovrd=off  show_param=off
      settings: xl_area=[0, 0, 0, 0, 0, 0, 0]
  data_FWFT : Subsystem  mask{depth_bits=depth_data_bits}
      mask prompts: depth_bits "Fifo Depth (2^?):"
      mask help: A rollback fifo behaves as a normal fifo, except that data which are written in have to be "committed" before they become available for readout. Moreover, any data which are written in and have not been committed can be "discarded", and will never be made available for readout.
      mask init:
      | fmtstr = sprintf('Depth: %d', 2^depth_bits);
      | set_param(gcb, 'AttributesFormatString', fmtstr);
      settings: AttributesFormatString=Depth: 1024
  data_debug : Scope  NumInputPorts=10
      settings: YMin=12000~0~9500~0~15500~0~0~-5~-5~-5  YMax=13300~1~10500~1~17250~1~1~5~5~5  SaveName=ScopeData8
  fifo_empty : xbsIndex_r3/Logical  logical_function=AND  inputs=2  precision=Full  arith_type=Unsigned  n_bits=8  bin_pt=2  align_bp=on  latency=0  explicit_period=off  period=1  en=off  dbl_ovrd=off  show_param=off
      settings: xl_area=[0, 0, 0, 0, 0, 0, 0]
  fifo_full : xbsIndex_r3/Logical  logical_function=OR  inputs=2  precision=Full  arith_type=Unsigned  n_bits=8  bin_pt=2  align_bp=on  latency=0  explicit_period=off  period=1  en=off  dbl_ovrd=off  show_param=off
      settings: xl_area=[0, 0, 0, 0, 0, 0, 0]
  ip_debug : Scope  NumInputPorts=6
      settings: YMin=100~0~0~100~0~-5  YMax=103~1~1~103~1~5  SaveName=ScopeData9
  ip_fifo : Subsystem  mask{depth_bits=depth_hdr_bits}
      mask prompts: depth_bits "Fifo Depth (2^?):"
      mask help: A rollback fifo behaves as a normal fifo, except that data which are written in have to be "committed" before they become available for readout. Moreover, any data which are written in and have not been committed can be "discarded", and will never be made available for readout.
      mask init:
      | fmtstr = sprintf('Depth: %d', 2^depth_bits);
      | set_param(gcb, 'AttributesFormatString', fmtstr);
      settings: AttributesFormatString=Depth: 32
  overflow_cnt : xps_library/software register  Tag=xps:sw_reg  io_dir=To Processor  arith_type=Unsigned  bitwidth=32  bin_pt=0  sample_period=1  gw_name=b_2x_8a_r310_a_xaui_buffer0_overflow_cnt_user_data_in
  overflows : xbsIndex_r3/Counter  cnt_type=Free Running  n_bits=32  bin_pt=0  arith_type=Unsigned  start_count=0  cnt_to=Inf  cnt_by_val=1  operation=Up  explicit_period=off  period=1  load_pin=off  rst=off  en=on  dbl_ovrd=off  show_param=off  use_rpm=on  gen_core=off
      settings: xl_area=[0, 0, 0, 0, 0, 0, 0]
  status : xps_library/software register  Tag=xps:sw_reg  io_dir=To Processor  arith_type=Unsigned  bitwidth=32  bin_pt=0  sample_period=1  gw_name=b_2x_8a_r310_a_xaui_buffer0_status_user_data_in
  status1 : Scope  NumInputPorts=4
      settings: YMin=-1~-1~-1~-1  YMax=1~1~1~1  SaveName=ScopeData6
  valid_eof_0 : xbsIndex_r3/Logical  logical_function=AND  inputs=2  precision=Full  arith_type=Unsigned  n_bits=8  bin_pt=2  align_bp=on  latency=0  explicit_period=on  period=1  en=off  dbl_ovrd=off  show_param=off
      settings: xl_area=[0, 0, 0, 0, 0, 0, 0]
  data : Outport
  valid : Outport  Port=2
  ip_addr : Outport  Port=3
  eof : Outport  Port=4
  discard : Outport  Port=5
  buffer_overflow : Outport  Port=6
  buffer_empty : Outport  Port=7
  ack_in : Outport  Port=8
  status_out : Outport  Port=9
  wires:
  Constant13/1 -> discard/1
  fifo_full/1 -> buffer_overflow/1, overflows/1
  fifo_empty/1 -> buffer_empty/1
  [ip_empty] -> fifo_empty/1
  [data_empty] -> fifo_empty/2
  [ip_full] -> fifo_full/1
  [data_full] -> fifo_full/2
  [ip_full] -> Convert1/1, Gateway Out7/1
  [data_full] -> Gateway Out8/1, Convert5/1
  [ip_empty] -> Convert8/1, Gateway Out6/1
  [data_empty] -> Convert9/1, Gateway Out14/1
  Concat_status/1 -> Concat3/2, status_out/1
  Concat3/1 -> status/1
  Constant7/1 -> Concat3/1
  discard_in/1 -> Convert3/1
  Concat/1 -> data_FWFT/1(din)
  data_FWFT/4(full) -> [data_full]
  ip_fifo/3(full) -> [ip_full]
  commit/1 -> ip_fifo/3(commit), ip_fifo/2(we), [ip_commit]
  d_in/1 -> Reinterpret/1
  valid_in/1 -> Convert/1
  dest_ip_0/1 -> ip_fifo/1(din), [ip_in]
  eof_in/1 -> Convert2/1
  data_FWFT/3(wr_ack) -> ack_in/1
  ip_fifo/4(empty) -> [ip_empty]
  Inverter4/1 -> commit/2
  valid_eof_0/1 -> Concat/1, [in_valid_eof], data_FWFT/3(commit)
  data_FWFT/1(dout) -> buf_eof1/1, buf_eof3/1, buf_data3/1
  data_FWFT/2(valid) -> valid/1, [v_out]
  ip_fifo/1(dout) -> ip_addr/1, [ip_out]
  Constant9/1 -> ip_fifo/4(discard)
  overflows/1 -> overflow_cnt/1
  Gateway Out24/1 -> data_debug/1
  Gateway Out22/1 -> data_debug/2
  Gateway Out23/1 -> data_debug/3
  Gateway Out25/1 -> data_debug/4
  Gateway Out29/1 -> ip_debug/1
  Gateway Out27/1 -> ip_debug/2
  Gateway Out28/1 -> ip_debug/3
  Gateway Out30/1 -> ip_debug/4
  Gateway Out31/1 -> ip_debug/5
  Gateway Out39/1 -> data_debug/5
  Gateway Out41/1 -> data_debug/6
  Gateway Out40/1 -> data_debug/7
  Gateway Out42/1 -> ip_debug/6
  data_FWFT/5(empty) -> [data_empty]
  buf_data3/1 -> data/1, [d_out]
  buf_eof3/1 -> eof/1, [eof_out]
  [in_valid_eof] -> commit/1
  Gateway Out7/1 -> status1/1
  Gateway Out8/1 -> status1/2
  Gateway Out6/1 -> status1/3
  Gateway Out14/1 -> status1/4
  Convert1/1 -> Concat_status/1
  Convert5/1 -> Concat_status/2
  Convert8/1 -> Concat_status/3
  Convert9/1 -> Concat_status/4
  Gateway Out1/1 -> data_debug/8
  [ip_out] -> Gateway Out1/1
  [eof_out] -> Gateway Out40/1
  [v_out] -> Gateway Out41/1
  [d_out] -> Gateway Out39/1
  [ip_in] -> Gateway Out25/1
  [d_in] -> Gateway Out24/1
  [v_in] -> Gateway Out22/1
  [in_valid_eof] -> Gateway Out23/1
  [ip_in] -> Gateway Out29/1
  [ip_out] -> Gateway Out30/1
  [eof_out] -> Gateway Out31/1
  ack_out/1 -> Convert4/1
  [data_ack] -> Gateway Out42/1
  [ip_commit] -> Gateway Out27/1
  [data_full] -> Inverter4/1
  [ip_fetch] -> Gateway Out28/1
  [data_ack] -> data_FWFT/5(ack)
  Gateway Out2/1 -> data_debug/9
  [data_ack] -> Gateway Out2/1
  buf_eof1/1 -> [ip_fetch]
  [ip_fetch] -> ip_fifo/5(fetch)
  Reinterpret/1 -> Concat/2, [d_in]
  Convert/1 -> valid_eof_0/1, [v_in], data_FWFT/2(we)
  Convert2/1 -> valid_eof_0/2
  Convert3/1 -> data_FWFT/4(discard)
  Convert4/1 -> [data_ack]
  Gateway Out3/1 -> data_debug/10
  [data_full] -> Gateway Out3/1

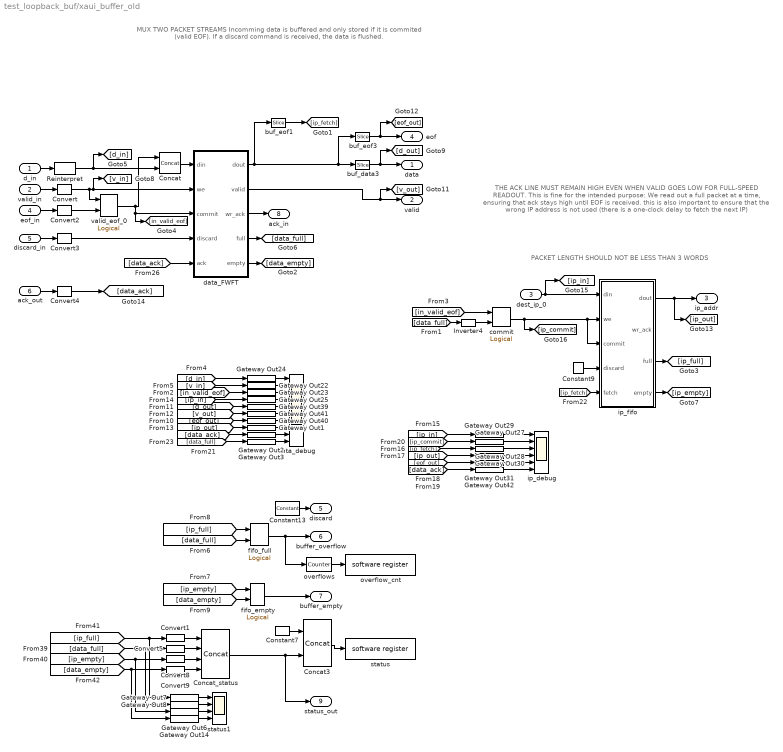
== system test_loopback_buf/xaui_buffer_old ==
  note: MUX TWO PACKET STREAMS
      | Incomming data is buffered and only stored if it is commited (valid EOF).
      | If a discard command is received, the data is flushed.
  note: THE ACK LINE MUST REMAIN HIGH EVEN WHEN VALID GOES LOW FOR FULL-SPEED READOUT.
      |
      | This is fine for the intended purpose:
      | We read out a full packet at a time, ensuring that ack stays high until EOF is received.
      |
      | this is also important to ensure that the wrong IP address is not used
      | (there is a one-clock delay to fetch the next IP)
  note: PACKET LENGTH SHOULD NOT BE LESS THAN 3 WORDS
  d_in : Inport  Port=1  LatchInput=off
  valid_in : Inport  Port=2  LatchInput=off
  dest_ip_0 : Inport  Port=3  LatchInput=off
  eof_in : Inport  Port=4  LatchInput=off
  discard_in : Inport  Port=5  LatchInput=off
  ack_out : Inport  Port=6  LatchInput=off
  Concat : xbsIndex_r3/Concat  num_inputs=2  explicit_period=off  period=1  dbl_ovrd=off
  Concat3 : xbsIndex_r3/Concat  num_inputs=2  explicit_period=off  period=1  dbl_ovrd=off
  Concat_status : xbsIndex_r3/Concat  num_inputs=4  explicit_period=on  period=1  dbl_ovrd=off
  Constant13 : xbsIndex_r3/Constant  const=0  equ=P=C  arith_type=Boolean  n_bits=1  bin_pt=0  opselect=C  inp2=PCIN>>17  opr=+  inp1=P  carry=CIN  iostate=0  explicit_period=on  period=1  dbl_ovrd=off
  Constant7 : xbsIndex_r3/Constant  const=0  equ=P=C  arith_type=Unsigned  n_bits=32-9  bin_pt=0  opselect=C  inp2=PCIN>>17  opr=+  inp1=P  carry=CIN  iostate=0  explicit_period=on  period=1  dbl_ovrd=off
  Constant9 : xbsIndex_r3/Constant  const=0  equ=P=C  arith_type=Boolean  n_bits=1  bin_pt=0  opselect=C  inp2=PCIN>>17  opr=+  inp1=P  carry=CIN  iostate=0  explicit_period=on  period=1  dbl_ovrd=off
  Convert{,2..4} (4 alike) : xbsIndex_r3/Convert  arith_type=Boolean  n_bits=8  bin_pt=6  quantization=Truncate  overflow=Wrap  latency=0  explicit_period=on  period=1  dbl_ovrd=off  show_param=off  inserted_by_tool=off  pipeline=off
      settings: xl_area=[0, 0, 0, 0, 0, 0, 0]
  Convert{1,5,8..9} (4 alike) : xbsIndex_r3/Convert  arith_type=Unsigned  n_bits=1  bin_pt=0  quantization=Truncate  overflow=Wrap  latency=0  explicit_period=off  period=1  dbl_ovrd=off  show_param=off  inserted_by_tool=off  pipeline=off
      settings: xl_area=[0, 0, 0, 0, 0, 0, 0]
  Gateway Out{1..3,6..8,14,22..25,27..31,39..42} (20 alike) : xbsIndex_r3/Gateway Out  output_type=Double  nbits=8  bin_pt=6  arith_type=Boolean  quantization=Truncate  overflow=Wrap  hdl_port=on  timing_constraint=None  locs_specified=off  LOCs={}  needs_fixed_name=off  show_param=off
      settings: xl_area=[0, 0, 0, 0, 0, 0, 0]
  Inverter4 : xbsIndex_r3/Inverter  latency=0  explicit_period=off  period=1  en=off  dbl_ovrd=off  show_param=off
      settings: xl_area=[0, 0, 0, 0, 0, 0, 0]
  Reinterpret : xbsIndex_r3/Reinterpret  force_arith_type=on  arith_type=Unsigned  force_bin_pt=on  bin_pt=0  force_valid=on
  buf_data3 : xbsIndex_r3/Slice  mode=Lower Bit Location + Width  nbits=64  bit1=33  base1=LSB of Input  bit0=0  base0=LSB of Input  boolean_output=off  explicit_period=off  period=1  dbl_ovrd=off
  buf_eof1 : xbsIndex_r3/Slice  mode=Upper Bit Location + Width  nbits=1  bit1=64  base1=LSB of Input  bit0=0  base0=LSB of Input  boolean_output=on  explicit_period=off  period=1  dbl_ovrd=off
  buf_eof3 : xbsIndex_r3/Slice  mode=Upper Bit Location + Width  nbits=1  bit1=64  base1=LSB of Input  bit0=0  base0=LSB of Input  boolean_output=on  explicit_period=off  period=1  dbl_ovrd=off
  commit : xbsIndex_r3/Logical  logical_function=AND  inputs=2  precision=Full  arith_type=Unsigned  n_bits=8  bin_pt=2  align_bp=on  latency=0  explicit_period=off  period=1  en=off  dbl_ovrd=off  show_param=off
      settings: xl_area=[0, 0, 0, 0, 0, 0, 0]
  data_FWFT : Subsystem  mask{depth_bits=depth_data_bits}
      mask prompts: depth_bits "Fifo Depth (2^?):"
      mask help: A rollback fifo behaves as a normal fifo, except that data which are written in have to be "committed" before they become available for readout. Moreover, any data which are written in and have not been committed can be "discarded", and will never be made available for readout.
      mask init:
      | fmtstr = sprintf('Depth: %d', 2^depth_bits);
      | set_param(gcb, 'AttributesFormatString', fmtstr);
      settings: AttributesFormatString=Depth: 1024
  data_debug : Scope  NumInputPorts=10
      settings: YMin=12000~0~9500~0~15500~0~0~-5~-5~-5  YMax=13300~1~10500~1~17250~1~1~5~5~5  SaveName=ScopeData8
  fifo_empty : xbsIndex_r3/Logical  logical_function=AND  inputs=2  precision=Full  arith_type=Unsigned  n_bits=8  bin_pt=2  align_bp=on  latency=0  explicit_period=off  period=1  en=off  dbl_ovrd=off  show_param=off
      settings: xl_area=[0, 0, 0, 0, 0, 0, 0]
  fifo_full : xbsIndex_r3/Logical  logical_function=OR  inputs=2  precision=Full  arith_type=Unsigned  n_bits=8  bin_pt=2  align_bp=on  latency=0  explicit_period=off  period=1  en=off  dbl_ovrd=off  show_param=off
      settings: xl_area=[0, 0, 0, 0, 0, 0, 0]
  ip_debug : Scope  NumInputPorts=6
      settings: YMin=100~0~0~100~0~-5  YMax=103~1~1~103~1~5  SaveName=ScopeData9
  ip_fifo : Subsystem  mask{depth_bits=depth_hdr_bits}
      mask prompts: depth_bits "Fifo Depth (2^?):"
      mask help: A rollback fifo behaves as a normal fifo, except that data which are written in have to be "committed" before they become available for readout. Moreover, any data which are written in and have not been committed can be "discarded", and will never be made available for readout.
      mask init:
      | fmtstr = sprintf('Depth: %d', 2^depth_bits);
      | set_param(gcb, 'AttributesFormatString', fmtstr);
      settings: AttributesFormatString=Depth: 256
  overflow_cnt : xps_library/software register  Tag=xps:sw_reg  io_dir=To Processor  arith_type=Unsigned  bitwidth=32  bin_pt=0  sample_period=1  gw_name=test_loopback_buf_xaui_buffer_old_overflow_cnt_user_data_in
  overflows : xbsIndex_r3/Counter  cnt_type=Free Running  n_bits=32  bin_pt=0  arith_type=Unsigned  start_count=0  cnt_to=Inf  cnt_by_val=1  operation=Up  explicit_period=off  period=1  load_pin=off  rst=off  en=on  dbl_ovrd=off  show_param=off  use_rpm=on  gen_core=off
      settings: xl_area=[0, 0, 0, 0, 0, 0, 0]
  status : xps_library/software register  Tag=xps:sw_reg  io_dir=To Processor  arith_type=Unsigned  bitwidth=32  bin_pt=0  sample_period=1  gw_name=test_loopback_buf_xaui_buffer_old_status_user_data_in
  status1 : Scope  NumInputPorts=4
      settings: YMin=-1~-1~-1~-1  YMax=1~1~1~1  SaveName=ScopeData6
  valid_eof_0 : xbsIndex_r3/Logical  logical_function=AND  inputs=2  precision=Full  arith_type=Unsigned  n_bits=8  bin_pt=2  align_bp=on  latency=0  explicit_period=on  period=1  en=off  dbl_ovrd=off  show_param=off
      settings: xl_area=[0, 0, 0, 0, 0, 0, 0]
  data : Outport
  valid : Outport  Port=2
  ip_addr : Outport  Port=3
  eof : Outport  Port=4
  discard : Outport  Port=5
  buffer_overflow : Outport  Port=6
  buffer_empty : Outport  Port=7
  ack_in : Outport  Port=8
  status_out : Outport  Port=9
  wires:
  Constant13/1 -> discard/1
  fifo_full/1 -> buffer_overflow/1, overflows/1
  fifo_empty/1 -> buffer_empty/1
  [ip_empty] -> fifo_empty/1
  [data_empty] -> fifo_empty/2
  [ip_full] -> fifo_full/1
  [data_full] -> fifo_full/2
  [ip_full] -> Convert1/1, Gateway Out7/1
  [data_full] -> Gateway Out8/1, Convert5/1
  [ip_empty] -> Convert8/1, Gateway Out6/1
  [data_empty] -> Convert9/1, Gateway Out14/1
  Concat_status/1 -> Concat3/2, status_out/1
  Concat3/1 -> status/1
  Constant7/1 -> Concat3/1
  discard_in/1 -> Convert3/1
  Concat/1 -> data_FWFT/1(din)
  data_FWFT/4(full) -> [data_full]
  ip_fifo/3(full) -> [ip_full]
  commit/1 -> ip_fifo/3(commit), ip_fifo/2(we), [ip_commit]
  d_in/1 -> Reinterpret/1
  valid_in/1 -> Convert/1
  dest_ip_0/1 -> ip_fifo/1(din), [ip_in]
  eof_in/1 -> Convert2/1
  data_FWFT/3(wr_ack) -> ack_in/1
  ip_fifo/4(empty) -> [ip_empty]
  Inverter4/1 -> commit/2
  valid_eof_0/1 -> Concat/1, [in_valid_eof], data_FWFT/3(commit)
  data_FWFT/1(dout) -> buf_eof1/1, buf_eof3/1, buf_data3/1
  data_FWFT/2(valid) -> valid/1, [v_out]
  ip_fifo/1(dout) -> ip_addr/1, [ip_out]
  Constant9/1 -> ip_fifo/4(discard)
  overflows/1 -> overflow_cnt/1
  Gateway Out24/1 -> data_debug/1
  Gateway Out22/1 -> data_debug/2
  Gateway Out23/1 -> data_debug/3
  Gateway Out25/1 -> data_debug/4
  Gateway Out29/1 -> ip_debug/1
  Gateway Out27/1 -> ip_debug/2
  Gateway Out28/1 -> ip_debug/3
  Gateway Out30/1 -> ip_debug/4
  Gateway Out31/1 -> ip_debug/5
  Gateway Out39/1 -> data_debug/5
  Gateway Out41/1 -> data_debug/6
  Gateway Out40/1 -> data_debug/7
  Gateway Out42/1 -> ip_debug/6
  data_FWFT/5(empty) -> [data_empty]
  buf_data3/1 -> data/1, [d_out]
  buf_eof3/1 -> eof/1, [eof_out]
  [in_valid_eof] -> commit/1
  Gateway Out7/1 -> status1/1
  Gateway Out8/1 -> status1/2
  Gateway Out6/1 -> status1/3
  Gateway Out14/1 -> status1/4
  Convert1/1 -> Concat_status/1
  Convert5/1 -> Concat_status/2
  Convert8/1 -> Concat_status/3
  Convert9/1 -> Concat_status/4
  Gateway Out1/1 -> data_debug/8
  [ip_out] -> Gateway Out1/1
  [eof_out] -> Gateway Out40/1
  [v_out] -> Gateway Out41/1
  [d_out] -> Gateway Out39/1
  [ip_in] -> Gateway Out25/1
  [d_in] -> Gateway Out24/1
  [v_in] -> Gateway Out22/1
  [in_valid_eof] -> Gateway Out23/1
  [ip_in] -> Gateway Out29/1
  [ip_out] -> Gateway Out30/1
  [eof_out] -> Gateway Out31/1
  ack_out/1 -> Convert4/1
  [data_ack] -> Gateway Out42/1
  [ip_commit] -> Gateway Out27/1
  [data_full] -> Inverter4/1
  [ip_fetch] -> Gateway Out28/1
  [data_ack] -> data_FWFT/5(ack)
  Gateway Out2/1 -> data_debug/9
  [data_ack] -> Gateway Out2/1
  buf_eof1/1 -> [ip_fetch]
  [ip_fetch] -> ip_fifo/5(fetch)
  Reinterpret/1 -> Concat/2, [d_in]
  Convert/1 -> valid_eof_0/1, data_FWFT/2(we), [v_in]
  Convert2/1 -> valid_eof_0/2
  Convert3/1 -> data_FWFT/4(discard)
  Convert4/1 -> [data_ack]
  Gateway Out3/1 -> data_debug/10
  [data_full] -> Gateway Out3/1
